simulink model "qbmove_example_compatible"  (Simulink 8.1)
settings: Solver=ode1  StartTime=0.0  StopTime=2  FixedStep=0.0035  RelTol=1e-3
libraries: simulink x2, qbmove_library x2, QB_pacer_lib x1
settings Model: Creator=laurentio  LastModifiedBy=laurentio
settings DataIOCC: SignalLoggingSaveFormat=Dataset
settings OptimizationCC: ExpressionDepthLimit=128
settings DebuggingCC: FcnCallInpInsideContextMsg=EnableAllAsError
settings GRTTargetCC: CombineOutputUpdateFcns=on  GRTInterface=off

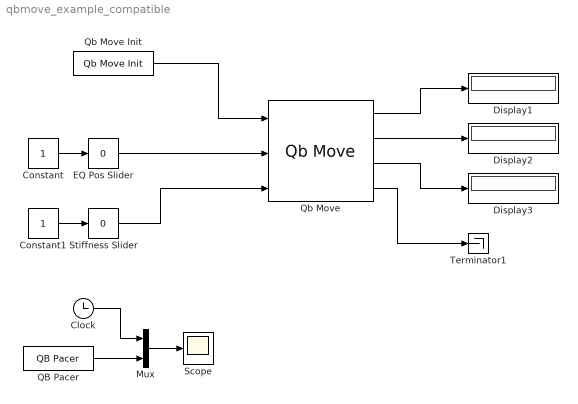
== system qbmove_example_compatible ==
  Clock : Clock
  Constant : Constant
  Constant1 : Constant
  Display1 : Display
  Display2 : Display
  Display3 : Display
  "EQ Pos Slider " : simulink/Math Operations/Slider Gain  low=-180  gain=0  high=180
  Mux : Mux  Inputs=2
  QB Pacer : QB_pacer_lib/QB Pacer  simTimePerRealTime=1
  Qb Move : qbmove_library/Qb Move  ID=3  ACTIVE_COMM_DIRECTIONS=Both  CONTROL_MODE=Equilibrium Position and Stiffness Preset  DAISY_CHAINING=off  MAX_ANG=0  SW_LIMIT=inf  OFFSET=0
  Qb Move Init : qbmove_library/Qb Move Init  NUMBER_OF_COM='/dev/ttyUSB0'
  Scope : Scope
      settings: YMin=0  YMax=5.5
  Stiffness Slider : simulink/Math Operations/Slider Gain  low=0  gain=0  high=30
  Terminator1 : Terminator
  wires:
  Qb Move Init/1 -> Qb Move/1
  Qb Move/1 -> Display1/1
  Qb Move/2 -> Display2/1
  Constant/1 -> "EQ Pos Slider "/1
  "EQ Pos Slider "/1 -> Qb Move/2
  Constant1/1 -> Stiffness Slider/1
  Stiffness Slider/1 -> Qb Move/3
  Qb Move/3 -> Display3/1
  QB Pacer/1 -> Mux/2
  Qb Move/4 -> Terminator1/1
  Clock/1 -> Mux/1
  Mux/1 -> Scope/1
